simulink model "verify_StorageTnodes_inverseTC_mdl"  (R2016b)
settings: Solver=ode45  StartTime=0.0  StopTime=1  MaxStep=60  RelTol=1e-3  EnableMultiTasking=on
libraries: carnot x3
settings Model: Creator=drhf  LastModifiedBy=drhf
settings DataIOCC: SaveFormat=Array  SignalLoggingSaveFormat=ModelDataLogs
settings OptimizationCC: ExpressionDepthLimit=2147483647  LifeSpan=inf
settings DebuggingCC: UnderspecifiedInitializationDetection=Classic  MergeDetectMultiDrivingBlocksExec=none  SolverPrmCheckMsg=warning  FcnCallInpInsideContextMsg=warning  StateNameClashWarn=warning  SFUnexpectedBacktrackingDiag=warning  SFNoUnconditionalDefaultTransitionDiag=warning  SFExecutionAtInitializationDiag=none
settings HardwareCC: ProdBitPerPointer=32  ProdBitPerSizeT=32  ProdBitPerPtrDiffT=32  ProdLargestAtomicFloat=None  ProdIntDivRoundTo=Undefined  ProdEndianess=Unspecified  ProdWordSize=32  ProdHWDeviceType=32-bit Generic
settings ModelReferenceCC: PropagateSignalLabelsOutOfModel=off
settings GRTTargetCC: TargetLangStandard=C89/C90 (ANSI)  GeneratePreprocessorConditionals=Disable all  CombineOutputUpdateFcns=off  GRTInterface=on
settings ConfigComp: CovMetricSettings=dw  CovHtmlReporting=on  CovSaveCumulativeToWorkspaceVar=on  CovSaveSingleToWorkspaceVar=on  CovExternalEMLEnable=off

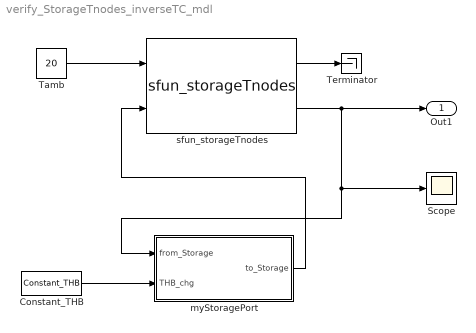
== system verify_StorageTnodes_inverseTC_mdl ==
  Constant_THB : carnot/Source/Simple/Constant_THB  t=40  mdot=0  p=1e5  mID=No Pressure Drop  fluid=Water (Constant 20°C)  mix=0  mix2=0  mix3=0  dia=0.02  hgt=0
  Scope : Scope
  Tamb : Constant  Value=20
  Terminator : Terminator
  myStoragePort : Subsystem  mask(Multiport Storage){uloss=1, ubot=1, utop=1, cond=1, t0=20, volume=1, dia=0.6, pos=standing cylinder, nconnect=1, nodes=10, mpoints=10}
      mask prompts: uloss "Heat loss coefficient cylinder wall in W/(m²K)"; ubot "Heat loss coefficient bottom in W/(m²K)"; utop "Heat loss coefficient top cover in W/(m²K)"; cond "Effective vertical conductivity in W/(m*K)"; t0 "Initial temperature (vector or scalar) in °C"; volume "Volume in m³"; dia "Diameter in m"; pos "Position"; nconnect "Number of connections"; nodes "Number of nodes"; mpoints "Number of measurement points"
      mask help:
      | The volmue of the cylindrical storage is divided in a number "nodes" of horizontal slices (1xN-node model). For each node the energy balance equation is solved.
      | Look under mask to set the ports types and properties.
      mask init:
      | [standing, dh, height, mpts, tini] ...
      |     = CarnotCallbacks_StorageTypeN(pos, volume, dia, nodes, mpoints, t0);
      mask Help: eval('man(''storage_multiport'')')
      mask TypeOptions pos: lying cylinder | standing cylinder
  sfun_storageTnodes : carnot/Basic/Thermal_Models/sfun_storageTnodes  uloss=0  ubot=0  utop=0  cond=0  volume=1  dia=0.6  standing=standing cylinder  tini=[55:-5:10]  nodes=10  nconnect=1  elimthermocline=0  condinvtc=1e5
  Out1 : Outport
  wires:
  Tamb/1 -> sfun_storageTnodes/1
  myStoragePort/1(to_Storage) -> sfun_storageTnodes/2
  sfun_storageTnodes/2 -> myStoragePort/1(from_Storage), Scope/1, Out1/1
  Constant_THB/1 -> myStoragePort/2(THB_chg)
  sfun_storageTnodes/1 -> Terminator/1

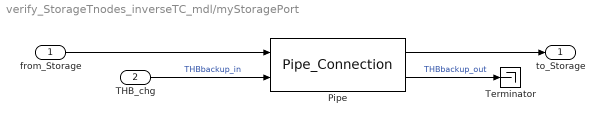
== system verify_StorageTnodes_inverseTC_mdl/myStoragePort ==
  from_Storage : Inport
  THB_chg : Inport  Port=2
  Pipe : carnot/Storage/Thermal/Storage_Ports/Pipe_Connection  h_in=1  h_out=0  hgt=1.0/(0.25*0.6^2*pi)  dia=0.6  height=-3.5368  nodes=nodes
  Terminator : Terminator
  to_Storage : Outport
  wires:
  THB_chg/1 -> Pipe/2  "THBbackup_in"
  from_Storage/1 -> Pipe/1
  Pipe/1 -> to_Storage/1
  Pipe/2 -> Terminator/1  "THBbackup_out"
